simulink model "CHW2_Q8_Simulink"  (R2021b)
settings: Solver=VariableStepAuto  StartTime=0.0  StopTime=10.0  RelTol=1e-3
settings Model: Creator=Matin  LastModifiedBy=Matin

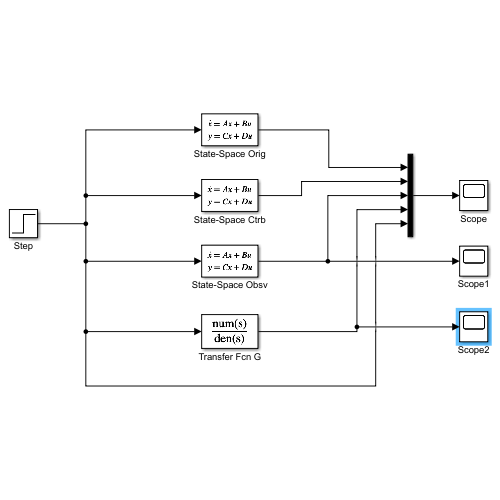
[thumbnail: Simulink's stored preview of the top-level diagram]
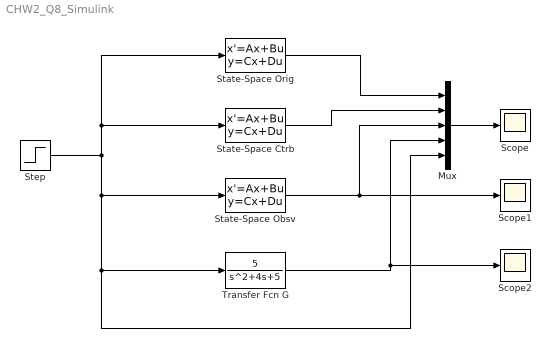
== system CHW2_Q8_Simulink ==
  Mux : Mux  Inputs=5
  Scope : Scope
  Scope1 : Scope
  Scope2 : Scope
  State-Space Ctrb : StateSpace  A=[0 -5; 1 -4]  B=[1;0]  C=[0 5]  D=0  InitialCondition=0
  State-Space Obsv : StateSpace  A=[-2 1;-1 -2]  B=[1.499;-5.646]  C=[-0.8273 -0.2197]  D=0  InitialCondition=0
  State-Space Orig : StateSpace  A=[-4 -2.5;2 0]  B=[2;0]  C=[0 1.25]  D=0  InitialCondition=0
  Step : Step  Time=0  SampleTime=0
  Transfer Fcn G : TransferFcn  Numerator=[0 0 5]  Denominator=[1 4 5]
  wires:
  Step/1 -> State-Space Ctrb/1, State-Space Orig/1, Mux/5, Transfer Fcn G/1, State-Space Obsv/1
  State-Space Ctrb/1 -> Mux/2
  State-Space Orig/1 -> Mux/1
  Transfer Fcn G/1 -> Scope2/1, Mux/4
  Mux/1 -> Scope/1
  State-Space Obsv/1 -> Scope1/1, Mux/3
